simulink model "gm_sampleModel1698_2_sub"  (R2023a)
settings: Solver=VariableStepAuto  StartTime=0.0  StopTime=10.0  RelTol=1e-3
libraries: simulink x1
settings Model: Creator=user1  LastModifiedBy=user1
settings OptimizationCC: BlockReduction=off  ConditionallyExecuteInputs=off
settings DebuggingCC: InheritedTsInSrcMsg=none

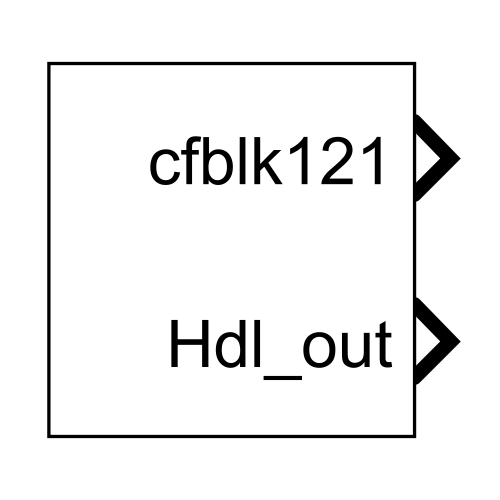
[thumbnail: Simulink's stored preview of the top-level diagram]
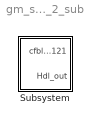
== system gm_sampleModel1698_2_sub ==
  Subsystem : Subsystem

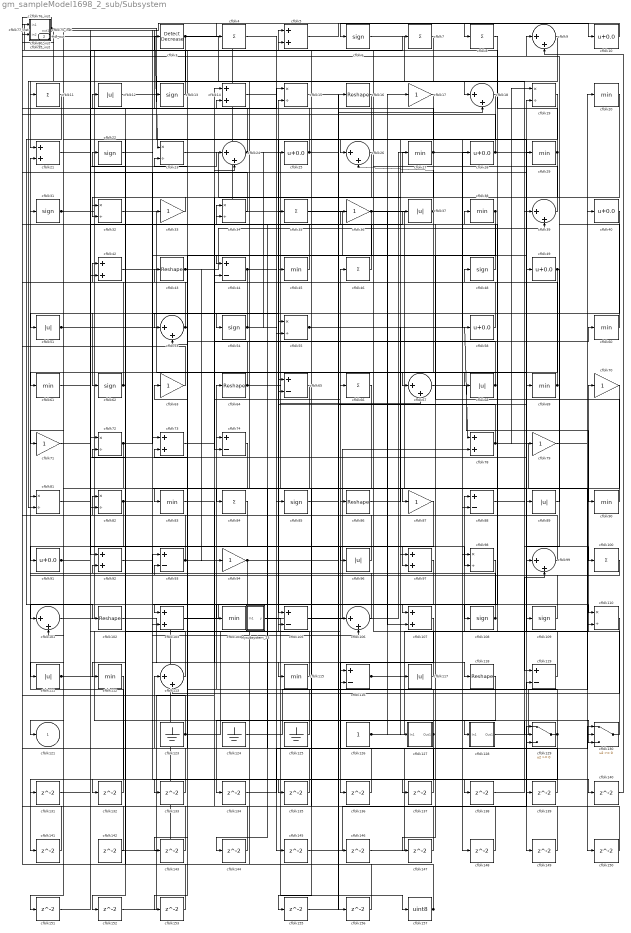
== system gm_sampleModel1698_2_sub/Subsystem ==
  Mysubsystem_23 : Subsystem
  cfblk{10,25,28,40,49,58,91} (7 alike) : Bias  Bias=0.0  SaturateOnIntegerOverflow=off
  cfblk{4,7..8,11,35,46,66,84,100} (9 alike) : Sum  Inputs=+  OutDataTypeStr=uint8
  cfblk{9,18,24,26,39,53,67,99,101,106,113} (11 alike) : Sum  Inputs=|++  OutDataTypeStr=uint8
  cfblk{16,43,64,86,102,118} (6 alike) : Reshape
  cfblk{5,14,21,42,73,78,92,97,103,107} (10 alike) : Sum  OutDataTypeStr=uint8
  cfblk{20,27,29,38,45,60..61,69,83,90,104,112,115} (13 alike) : MinMax  OutDataTypeStr=uint8
  cfblk{44,65,74,88,93,105,116,119} (8 alike) : Sum  Inputs=+-  OutDataTypeStr=uint8
  cfblk{6,13,22,31,48,54,62,85,108..109} (10 alike) : Signum
  cfblk{15,19,23,32,34,55,72,81..82,98,110} (11 alike) : Product  Inputs=*/  OutDataTypeStr=uint8  RndMeth=Zero  SaturateOnIntegerOverflow=on
  cfblk{12,37,51,68,89,96,111,117} (8 alike) : Abs  OutDataTypeStr=uint8  SaturateOnIntegerOverflow=off
  cfblk114_inst : Subsystem
  cfblk123 : Ground
  cfblk124 : Ground
  cfblk125 : Ground
  cfblk126 : Constant  OutDataTypeStr=uint8  SampleTime=-1
  cfblk127 : Subsystem
  cfblk128 : Subsystem
  cfblk129 : Switch  OutDataTypeStr=uint8  SaturateOnIntegerOverflow=off  InputSameDT=off
  cfblk130 : Switch  OutDataTypeStr=uint8  SaturateOnIntegerOverflow=off  InputSameDT=off
  cfblk{131..153,155..156} (25 alike) : Delay  SampleTime=1
  cfblk157 : DataTypeConversion  OutDataTypeStr=uint8  SaturateOnIntegerOverflow=off  RndMeth=Floor
  cfblk{17,33,36,63,70..71,79,87,94} (9 alike) : Gain  OutDataTypeStr=uint8
  cfblk2 : Constant  Value=0  OutDataTypeStr=uint8  SampleTime=1
  cfblk3 : simulink/Logic and Bit Operations/Detect Decrease  vinit=0.0  OutDataTypeStr=uint8
      settings: LibrarySourceBlock=|
      | hdlsllib/Logic and Bit
      | Operations/Detect
      | Decrease
  cfblk30_inst : Subsystem
  cfblk41_inst : Subsystem
  cfblk47_inst : Subsystem
  cfblk50_inst : Subsystem
  cfblk52_inst : Subsystem
  cfblk56_inst : Subsystem
  cfblk57_inst : Subsystem
  cfblk59_inst : Subsystem
  cfblk75_inst : Subsystem
  cfblk76_inst : Subsystem
  cfblk77_inst : Subsystem
  cfblk80_inst : Subsystem
  cfblk95_inst : Subsystem
  cfblk121 : Outport  OutDataTypeStr=uint8  SampleTime=1  VectorParamsAs1DForOutWhenUnconnected=off
  Hdl_out : Outport  Port=2  OutDataTypeStr=uint8  SampleTime=1
  wires:
  Mysubsystem_23/1(y) -> cfblk157/1
  cfblk10/1 -> cfblk6/1
  cfblk100/1 -> cfblk93/2
  cfblk101/1 -> cfblk5/1
  cfblk102/1 -> cfblk115/1
  cfblk103/1 -> cfblk107/1
  cfblk104/1 -> cfblk142/1
  cfblk105/1 -> cfblk78/2
  cfblk106/1 -> cfblk46/1
  cfblk107/1 -> cfblk136/1
  cfblk108/1 -> cfblk93/1, cfblk21/2
  cfblk109/1 -> cfblk31/1
  cfblk11/1 -> cfblk102/1
  cfblk110/1 -> cfblk113/2
  cfblk111/1 -> cfblk86/1, cfblk130/3
  cfblk112/1 -> cfblk141/1
  cfblk113/1 -> cfblk22/1
  cfblk114_inst/1(out1) -> cfblk23/1, cfblk149/1, cfblk148/1
  cfblk115/1 -> cfblk63/1
  cfblk116/1 -> cfblk70/1, cfblk19/2
  cfblk117/1 -> cfblk47_inst/1(in1)
  cfblk118/1 -> cfblk134/1
  cfblk119/1 -> cfblk38/1
  cfblk12/1 -> cfblk18/1
  cfblk123/1 -> cfblk77_inst/1(in1), cfblk15/2
  cfblk124/1 -> cfblk119/2
  cfblk125/1 -> cfblk56_inst/2(in2)
  cfblk126/1 -> cfblk88/1, cfblk17/1, cfblk110/2
  cfblk127/1(Out1) -> cfblk53/2, cfblk132/1
  cfblk128/1(Out1) -> cfblk20/1
  cfblk129/1 -> cfblk64/1, cfblk23/2, cfblk135/1
  cfblk13/1 -> cfblk95_inst/1(in1)
  cfblk130/1 -> cfblk41_inst/1(in1)
  cfblk131/1 -> cfblk105/2
  cfblk132/1 -> cfblk81/1
  cfblk133/1 -> cfblk47_inst/2(in2)
  cfblk134/1 -> cfblk130/1
  cfblk135/1 -> cfblk73/2
  cfblk136/1 -> cfblk34/1
  cfblk137/1 -> cfblk113/1
  cfblk138/1 -> cfblk99/2
  cfblk139/1 -> cfblk106/1
  cfblk14/1 -> cfblk49/1
  cfblk140/1 -> cfblk9/2
  cfblk141/1 -> cfblk80_inst/2(in2)
  cfblk142/1 -> cfblk50_inst/1(in1)
  cfblk143/1 -> cfblk82/1
  cfblk144/1 -> cfblk44/2
  cfblk145/1 -> cfblk129/1
  cfblk146/1 -> cfblk129/3
  cfblk147/1 -> cfblk5/2
  cfblk148/1 -> cfblk52_inst/2(in2)
  cfblk149/1 -> cfblk42/1
  cfblk15/1 -> cfblk156/1
  cfblk150/1 -> cfblk92/2
  cfblk151/1 -> cfblk72/1
  cfblk152/1 -> cfblk24/2
  cfblk153/1 -> cfblk57_inst/1(in1)
  cfblk155/1 -> cfblk18/2
  cfblk156/1 -> cfblk74/1
  cfblk157/1 -> cfblk75_inst/2(in2), cfblk12/1
  cfblk16/1 -> cfblk152/1
  cfblk17/1 -> cfblk26/1
  cfblk18/1 -> cfblk105/1
  cfblk19/1 -> cfblk51/1
  cfblk2/1 -> cfblk75_inst/1(in1), cfblk30_inst/2(in2), cfblk21/1, cfblk117/1
  cfblk20/1 -> cfblk108/1
  cfblk21/1 -> cfblk15/1
  cfblk22/1 -> cfblk96/1
  cfblk23/1 -> cfblk127/1(In1)
  cfblk24/1 -> cfblk67/2, cfblk59_inst/2(in2), cfblk3/1
  cfblk25/1 -> cfblk16/1, cfblk14/2
  cfblk26/1 -> cfblk74/2
  cfblk27/1 -> cfblk76_inst/1(in1), cfblk32/2
  cfblk28/1 -> cfblk76_inst/2(in2), cfblk114_inst/2(in2)
  cfblk29/1 -> cfblk65/1, cfblk114_inst/1(in1), Mysubsystem_23/1(In1)
  cfblk3/1 -> cfblk39/1, cfblk81/2
  cfblk30_inst/1(out1) -> cfblk10/1
  cfblk31/1 -> cfblk98/2, cfblk27/1
  cfblk32/1 -> cfblk55/1
  cfblk33/1 -> cfblk32/1
  cfblk34/1 -> cfblk56_inst/1(in1)
  cfblk35/1 -> cfblk98/1
  cfblk36/1 -> cfblk88/2, cfblk107/2, cfblk84/1
  cfblk37/1 -> cfblk67/1, cfblk26/2, Hdl_out/1
  cfblk38/1 -> cfblk147/1, cfblk83/1
  cfblk39/1 -> cfblk13/1
  cfblk4/1 -> cfblk139/1
  cfblk40/1 -> cfblk62/1
  cfblk41_inst/1(out1) -> cfblk73/1, cfblk55/2
  cfblk42/1 -> cfblk109/1
  cfblk43/1 -> cfblk39/2, cfblk94/1
  cfblk44/1 -> cfblk85/1, cfblk71/1
  cfblk45/1 -> cfblk80_inst/1(in1)
  cfblk46/1 -> cfblk34/2
  cfblk47_inst/1(out1) -> cfblk89/1, cfblk101/2
  cfblk48/1 -> cfblk41_inst/2(in2)
  cfblk49/1 -> cfblk99/1, cfblk87/1
  cfblk5/1 -> cfblk8/1
  cfblk50_inst/1(out1) -> cfblk33/1, cfblk45/1
  cfblk51/1 -> cfblk146/1, cfblk145/1
  cfblk52_inst/1(out1) -> cfblk92/1
  cfblk53/1 -> cfblk77_inst/2(in2), cfblk133/1
  cfblk54/1 -> cfblk97/2, cfblk53/1, cfblk25/1
  cfblk55/1 -> cfblk78/1, cfblk28/1
  cfblk56_inst/1(out1) -> cfblk130/2
  cfblk57_inst/1(out1) -> cfblk110/1
  cfblk58/1 -> cfblk14/1
  cfblk59_inst/1(out1) -> cfblk104/1
  cfblk6/1 -> cfblk119/1
  cfblk60/1 -> cfblk52_inst/1(in1)
  cfblk61/1 -> cfblk7/1
  cfblk62/1 -> cfblk59_inst/1(in1), cfblk112/1
  cfblk63/1 -> cfblk30_inst/1(in1)
  cfblk64/1 -> cfblk97/1, cfblk50_inst/2(in2)
  cfblk65/1 -> cfblk151/1
  cfblk66/1 -> cfblk155/1
  cfblk67/1 -> cfblk90/1
  cfblk68/1 -> cfblk95_inst/2(in2), cfblk61/1
  cfblk69/1 -> cfblk48/1, cfblk36/1
  cfblk7/1 -> cfblk91/1
  cfblk70/1 -> cfblk144/1
  cfblk71/1 -> cfblk24/1
  cfblk72/1 -> cfblk129/2, cfblk121/1, cfblk29/1
  cfblk73/1 -> cfblk60/1
  cfblk74/1 -> cfblk82/2
  cfblk75_inst/1(out1) -> cfblk103/2
  cfblk76_inst/1(out1) -> cfblk116/2, cfblk11/1
  cfblk77_inst/1(out1) -> cfblk118/1
  cfblk78/1 -> cfblk65/2, cfblk19/1, cfblk150/1
  cfblk79/1 -> cfblk40/1
  cfblk8/1 -> cfblk68/1
  cfblk80_inst/1(out1) -> cfblk54/1
  cfblk81/1 -> cfblk37/1
  cfblk82/1 -> cfblk106/2, cfblk131/1
  cfblk83/1 -> cfblk116/1
  cfblk84/1 -> cfblk111/1
  cfblk85/1 -> cfblk69/1
  cfblk86/1 -> cfblk58/1
  cfblk87/1 -> cfblk103/1
  cfblk88/1 -> cfblk100/1
  cfblk89/1 -> cfblk9/1
  cfblk9/1 -> cfblk44/1
  cfblk90/1 -> cfblk35/1
  cfblk91/1 -> cfblk42/2, cfblk79/1
  cfblk92/1 -> cfblk128/1(In1)
  cfblk93/1 -> cfblk57_inst/2(in2), cfblk66/1
  cfblk94/1 -> cfblk101/1, cfblk138/1, cfblk137/1
  cfblk95_inst/1(out1) -> cfblk140/1, cfblk4/1
  cfblk96/1 -> cfblk72/2
  cfblk97/1 -> cfblk153/1
  cfblk98/1 -> cfblk143/1
  cfblk99/1 -> cfblk43/1

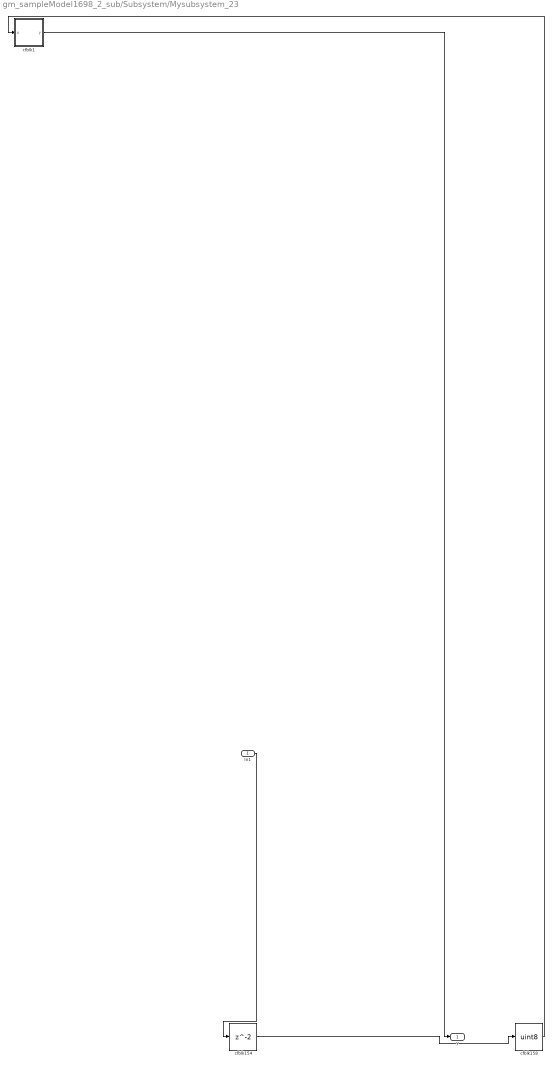
== system gm_sampleModel1698_2_sub/Subsystem/Mysubsystem_23 ==
  In1 : Inport  OutDataTypeStr=uint8  PortDimensions=1  SampleTime=1
  cfblk1 : Subsystem  mask(Compare To Zero){relop=<=, OutDataTypeStr=boolean, ZeroCross=on}
      mask prompts: relop "Simulink:masks:Operator_MP"; OutDataTypeStr "Simulink:masks:OutputDataType_MP"; ZeroCross "Simulink:masks:EnableZerocrossingDetection_MP"
      mask help: Simulink:masks:CompareToZero_MD
      mask init:
      | OutDataTypeStr = 'boolean';
      | ZeroCross = 'on';
      | blkName = 'sampleModel1698_2_sub/Subsystem/Mysubsystem_23/cfblk1';
      | relop = '<=';
      | setValue = 'boolean';
      mask TypeOptions relop: == | ~= | < | <= | >= | >
      mask TypeOptions OutDataTypeStr: Simulink:masks:uint8 | Simulink:masks:boolean
      mask Callback ZeroCross: sl('zeroCrossEnable', gcbh);
      mask Display: disp([relop,' 0'])
  cfblk154 : Delay  SampleTime=1
  cfblk158 : DataTypeConversion  OutDataTypeStr=uint8  SaturateOnIntegerOverflow=off  RndMeth=Floor
  y : Outport  SampleTime=1
  wires:
  In1/1 -> cfblk154/1
  cfblk1/1(y) -> y/1
  cfblk154/1 -> cfblk158/1
  cfblk158/1 -> cfblk1/1(u)

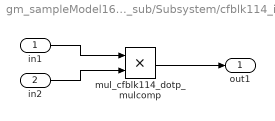
== system gm_sampleModel1698_2_sub/Subsystem/cfblk114_inst ==
  in1 : Inport  OutDataTypeStr=uint8  SampleTime=1
  in2 : Inport  Port=2  OutDataTypeStr=uint8  SampleTime=1
  mul_cfblk114_dotp_mulcomp : Product  Inputs=**  OutDataTypeStr=uint8  SampleTime=1
  out1 : Outport  OutDataTypeStr=uint8  SampleTime=1
  wires:
  in1/1 -> mul_cfblk114_dotp_mulcomp/1
  in2/1 -> mul_cfblk114_dotp_mulcomp/2
  mul_cfblk114_dotp_mulcomp/1 -> out1/1

== system gm_sampleModel1698_2_sub/Subsystem/cfblk127 ==
  In1 : Inport  OutDataTypeStr=uint8  PortDimensions=1  SampleTime=1
  Out1 : Outport  SampleTime=1
  wires:
  In1/1 -> Out1/1

== system gm_sampleModel1698_2_sub/Subsystem/cfblk128 ==
  In1 : Inport  OutDataTypeStr=uint8  PortDimensions=1  SampleTime=1
  Out1 : Outport  SampleTime=1
  wires:
  In1/1 -> Out1/1

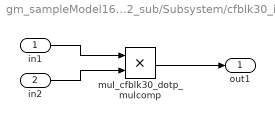
== system gm_sampleModel1698_2_sub/Subsystem/cfblk30_inst ==
  in1 : Inport  OutDataTypeStr=uint8  SampleTime=1
  in2 : Inport  Port=2  OutDataTypeStr=uint8  SampleTime=1
  mul_cfblk30_dotp_mulcomp : Product  Inputs=**  OutDataTypeStr=uint8  SampleTime=1
  out1 : Outport  OutDataTypeStr=uint8  SampleTime=1
  wires:
  in1/1 -> mul_cfblk30_dotp_mulcomp/1
  in2/1 -> mul_cfblk30_dotp_mulcomp/2
  mul_cfblk30_dotp_mulcomp/1 -> out1/1

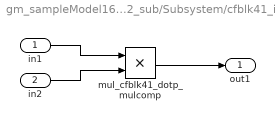
== system gm_sampleModel1698_2_sub/Subsystem/cfblk41_inst ==
  in1 : Inport  OutDataTypeStr=uint8  SampleTime=1
  in2 : Inport  Port=2  OutDataTypeStr=uint8  SampleTime=1
  mul_cfblk41_dotp_mulcomp : Product  Inputs=**  OutDataTypeStr=uint8  SampleTime=1
  out1 : Outport  OutDataTypeStr=uint8  SampleTime=1
  wires:
  in1/1 -> mul_cfblk41_dotp_mulcomp/1
  in2/1 -> mul_cfblk41_dotp_mulcomp/2
  mul_cfblk41_dotp_mulcomp/1 -> out1/1

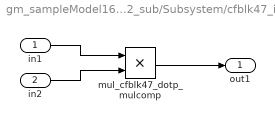
== system gm_sampleModel1698_2_sub/Subsystem/cfblk47_inst ==
  in1 : Inport  OutDataTypeStr=uint8  SampleTime=1
  in2 : Inport  Port=2  OutDataTypeStr=uint8  SampleTime=1
  mul_cfblk47_dotp_mulcomp : Product  Inputs=**  OutDataTypeStr=uint8  SampleTime=1
  out1 : Outport  OutDataTypeStr=uint8  SampleTime=1
  wires:
  in1/1 -> mul_cfblk47_dotp_mulcomp/1
  in2/1 -> mul_cfblk47_dotp_mulcomp/2
  mul_cfblk47_dotp_mulcomp/1 -> out1/1

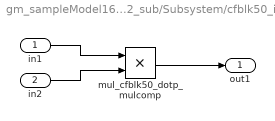
== system gm_sampleModel1698_2_sub/Subsystem/cfblk50_inst ==
  in1 : Inport  OutDataTypeStr=uint8  SampleTime=1
  in2 : Inport  Port=2  OutDataTypeStr=uint8  SampleTime=1
  mul_cfblk50_dotp_mulcomp : Product  Inputs=**  OutDataTypeStr=uint8  SampleTime=1
  out1 : Outport  OutDataTypeStr=uint8  SampleTime=1
  wires:
  in1/1 -> mul_cfblk50_dotp_mulcomp/1
  in2/1 -> mul_cfblk50_dotp_mulcomp/2
  mul_cfblk50_dotp_mulcomp/1 -> out1/1

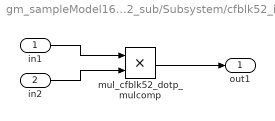
== system gm_sampleModel1698_2_sub/Subsystem/cfblk52_inst ==
  in1 : Inport  OutDataTypeStr=uint8  SampleTime=1
  in2 : Inport  Port=2  OutDataTypeStr=uint8  SampleTime=1
  mul_cfblk52_dotp_mulcomp : Product  Inputs=**  OutDataTypeStr=uint8  SampleTime=1
  out1 : Outport  OutDataTypeStr=uint8  SampleTime=1
  wires:
  in1/1 -> mul_cfblk52_dotp_mulcomp/1
  in2/1 -> mul_cfblk52_dotp_mulcomp/2
  mul_cfblk52_dotp_mulcomp/1 -> out1/1

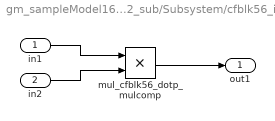
== system gm_sampleModel1698_2_sub/Subsystem/cfblk56_inst ==
  in1 : Inport  OutDataTypeStr=uint8  SampleTime=1
  in2 : Inport  Port=2  OutDataTypeStr=uint8  SampleTime=1
  mul_cfblk56_dotp_mulcomp : Product  Inputs=**  OutDataTypeStr=uint8  SampleTime=1
  out1 : Outport  OutDataTypeStr=uint8  SampleTime=1
  wires:
  in1/1 -> mul_cfblk56_dotp_mulcomp/1
  in2/1 -> mul_cfblk56_dotp_mulcomp/2
  mul_cfblk56_dotp_mulcomp/1 -> out1/1

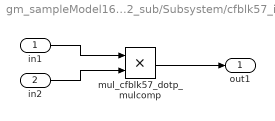
== system gm_sampleModel1698_2_sub/Subsystem/cfblk57_inst ==
  in1 : Inport  OutDataTypeStr=uint8  SampleTime=1
  in2 : Inport  Port=2  OutDataTypeStr=uint8  SampleTime=1
  mul_cfblk57_dotp_mulcomp : Product  Inputs=**  OutDataTypeStr=uint8  SampleTime=1
  out1 : Outport  OutDataTypeStr=uint8  SampleTime=1
  wires:
  in1/1 -> mul_cfblk57_dotp_mulcomp/1
  in2/1 -> mul_cfblk57_dotp_mulcomp/2
  mul_cfblk57_dotp_mulcomp/1 -> out1/1

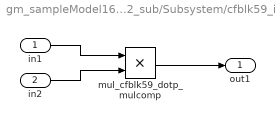
== system gm_sampleModel1698_2_sub/Subsystem/cfblk59_inst ==
  in1 : Inport  OutDataTypeStr=uint8  SampleTime=1
  in2 : Inport  Port=2  OutDataTypeStr=uint8  SampleTime=1
  mul_cfblk59_dotp_mulcomp : Product  Inputs=**  OutDataTypeStr=uint8  SampleTime=1
  out1 : Outport  OutDataTypeStr=uint8  SampleTime=1
  wires:
  in1/1 -> mul_cfblk59_dotp_mulcomp/1
  in2/1 -> mul_cfblk59_dotp_mulcomp/2
  mul_cfblk59_dotp_mulcomp/1 -> out1/1

== system gm_sampleModel1698_2_sub/Subsystem/cfblk75_inst ==
  in1 : Inport  OutDataTypeStr=uint8  SampleTime=1
  in2 : Inport  Port=2  OutDataTypeStr=uint8  SampleTime=1
  mul_cfblk75_dotp_mulcomp : Product  Inputs=**  OutDataTypeStr=uint8  SampleTime=1
  out1 : Outport  OutDataTypeStr=uint8  SampleTime=1
  wires:
  in1/1 -> mul_cfblk75_dotp_mulcomp/1
  in2/1 -> mul_cfblk75_dotp_mulcomp/2
  mul_cfblk75_dotp_mulcomp/1 -> out1/1

== system gm_sampleModel1698_2_sub/Subsystem/cfblk76_inst ==
  in1 : Inport  OutDataTypeStr=uint8  SampleTime=1
  in2 : Inport  Port=2  OutDataTypeStr=uint8  SampleTime=1
  mul_cfblk76_dotp_mulcomp : Product  Inputs=**  OutDataTypeStr=uint8  SampleTime=1
  out1 : Outport  OutDataTypeStr=uint8  SampleTime=1
  wires:
  in1/1 -> mul_cfblk76_dotp_mulcomp/1
  in2/1 -> mul_cfblk76_dotp_mulcomp/2
  mul_cfblk76_dotp_mulcomp/1 -> out1/1

== system gm_sampleModel1698_2_sub/Subsystem/cfblk77_inst ==
  in1 : Inport  OutDataTypeStr=uint8  SampleTime=1
  in2 : Inport  Port=2  OutDataTypeStr=uint8  SampleTime=1
  mul_cfblk77_dotp_mulcomp : Product  Inputs=**  OutDataTypeStr=uint8  SampleTime=1
  out1 : Outport  OutDataTypeStr=uint8  SampleTime=1
  wires:
  in1/1 -> mul_cfblk77_dotp_mulcomp/1
  in2/1 -> mul_cfblk77_dotp_mulcomp/2
  mul_cfblk77_dotp_mulcomp/1 -> out1/1

== system gm_sampleModel1698_2_sub/Subsystem/cfblk80_inst ==
  in1 : Inport  OutDataTypeStr=uint8  SampleTime=1
  in2 : Inport  Port=2  OutDataTypeStr=uint8  SampleTime=1
  mul_cfblk80_dotp_mulcomp : Product  Inputs=**  OutDataTypeStr=uint8  SampleTime=1
  out1 : Outport  OutDataTypeStr=uint8  SampleTime=1
  wires:
  in1/1 -> mul_cfblk80_dotp_mulcomp/1
  in2/1 -> mul_cfblk80_dotp_mulcomp/2
  mul_cfblk80_dotp_mulcomp/1 -> out1/1

== system gm_sampleModel1698_2_sub/Subsystem/cfblk95_inst ==
  in1 : Inport  OutDataTypeStr=uint8  SampleTime=1
  in2 : Inport  Port=2  OutDataTypeStr=uint8  SampleTime=1
  mul_cfblk95_dotp_mulcomp : Product  Inputs=**  OutDataTypeStr=uint8  SampleTime=1
  out1 : Outport  OutDataTypeStr=uint8  SampleTime=1
  wires:
  in1/1 -> mul_cfblk95_dotp_mulcomp/1
  in2/1 -> mul_cfblk95_dotp_mulcomp/2
  mul_cfblk95_dotp_mulcomp/1 -> out1/1

== system gm_sampleModel1698_2_sub/Subsystem/Mysubsystem_23/cfblk1 ==
  u : Inport  OutDataTypeStr=uint8  SampleTime=1
  Compare : RelationalOperator  Operator=<=  OutDataTypeStr=boolean
  Constant : Constant  DisableCoverage=on  Value=0  OutDataTypeStr=Inherit: Inherit via back propagation  SampleTime=-1  PreserveConstantTs=on
  y : Outport  SampleTime=1
  wires:
  u/1 -> Compare/1
  Compare/1 -> y/1
  Constant/1 -> Compare/2
